simulink model "lab2_2"  (R2022a)
settings: Solver=VariableStepAuto  StartTime=0.0  StopTime=10.0  RelTol=1e-3
settings Model: Creator=Комп  LastModifiedBy=Комп

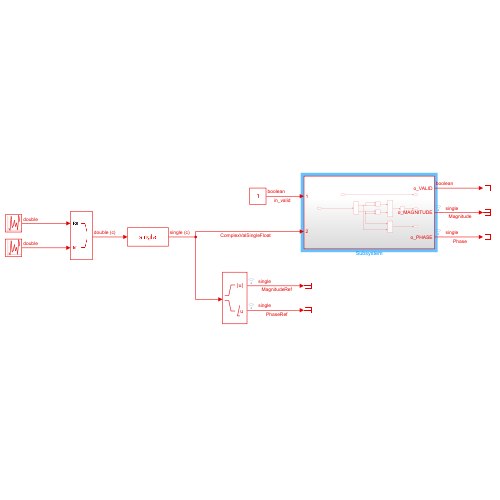
[thumbnail: Simulink's stored preview of the top-level diagram]
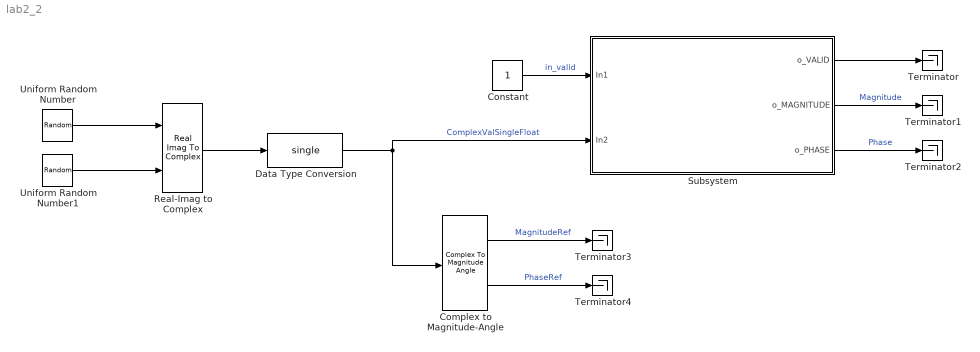
== system lab2_2 ==
  Complex to Magnitude-Angle : ComplexToMagnitudeAngle
  Constant : Constant  OutDataTypeStr=boolean  SampleTime=1
  Data Type Conversion : DataTypeConversion  OutDataTypeStr=single  RndMeth=Round  SaturateOnIntegerOverflow=off
  Real-Imag to Complex : RealImagToComplex
  Subsystem : Subsystem
  Terminator{,1..4} (5 alike) : Terminator
  Uniform Random Number : UniformRandomNumber  Minimum=0  Maximum=2^(18)-1  Seed=18  SampleTime=1
  Uniform Random Number1 : UniformRandomNumber  Minimum=0  Maximum=2^(18)-1  Seed=19  SampleTime=1
  wires:
  Uniform Random Number1/1 -> Real-Imag to Complex/2
  Uniform Random Number/1 -> Real-Imag to Complex/1
  Real-Imag to Complex/1 -> Data Type Conversion/1
  Data Type Conversion/1 -> Complex to Magnitude-Angle/1, Subsystem/2(In2)  "ComplexValSingleFloat"
  Complex to Magnitude-Angle/2 -> Terminator4/1  "PhaseRef"
  Complex to Magnitude-Angle/1 -> Terminator3/1  "MagnitudeRef"
  Constant/1 -> Subsystem/1(In1)  "in_valid"
  Subsystem/1(o_VALID) -> Terminator/1
  Subsystem/2(o_MAGNITUDE) -> Terminator1/1  "Magnitude"
  Subsystem/3(o_PHASE) -> Terminator2/1  "Phase"

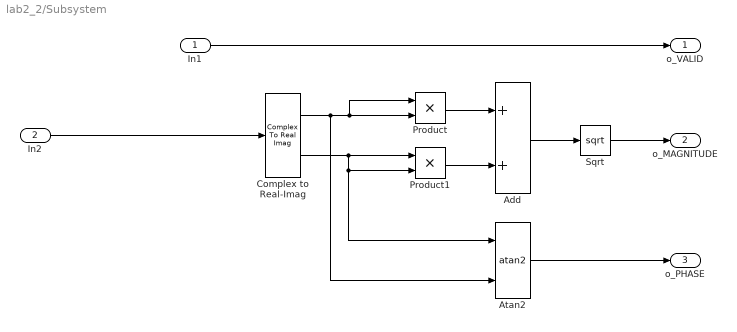
== system lab2_2/Subsystem ==
  In1 : Inport
  In2 : Inport  Port=2
  Add : Sum
  Atan2 : Trigonometry  Operator=atan2  ApproximationMethod=CORDIC
  Complex to Real-Imag : ComplexToRealImag
  Product : Product
  Product1 : Product
  Sqrt : Sqrt  OutDataTypeStr=Inherit: Inherit via internal rule
  o_VALID : Outport
  o_MAGNITUDE : Outport  Port=2
  o_PHASE : Outport  Port=3
  wires:
  Complex to Real-Imag/2 -> Atan2/1, Product1/2, Product1/1
  Add/1 -> Sqrt/1
  Complex to Real-Imag/1 -> Atan2/2, Product/1, Product/2
  Product1/1 -> Add/2
  Product/1 -> Add/1
  Sqrt/1 -> o_MAGNITUDE/1
  In2/1 -> Complex to Real-Imag/1
  In1/1 -> o_VALID/1
  Atan2/1 -> o_PHASE/1
